simulink model "SimulinkBallBallancingBeam(EA)"  (R2019b)
settings: Solver=FixedStepAuto  StartTime=0.0  StopTime=10  RelTol=1e-3  EnableMultiTasking=on
values from neighbouring files (symbols this model uses):
  d = 0.05    [BallBallancingBeam(EA).m]    (also in System_Parameters.m; TransferFunction.m)
  g = -9.81    [BallBallancingBeam(EA).m]    (also in System_Parameters.m; TransferFunction.m)
  J = 6.3e-7    (= 6.3e-07)    [BallBallancingBeam(EA).m]    (also in System_Parameters.m = 6.2e-07; TransferFunction.m = 6.2e-07)
  L = .4    (= 0.4)    [BallBallancingBeam(EA).m]    (also in System_Parameters.m = 0.2; TransferFunction.m = 0.2)
  m = 0.0027    [BallBallancingBeam(EA).m]    (also in System_Parameters.m; TransferFunction.m)
  R = 0.02    [BallBallancingBeam(EA).m]    (also in System_Parameters.m = 0.0201; TransferFunction.m = 0.0201)
libraries: arduinolib x4, simulink x2, arduinosensorlib x1
settings Model: SILPILModeSetting=veronly  ExtModeTrigDuration=2  Creator=erika  LastModifiedBy=erika
settings SolverCC: PositivePriorityOrder=on
settings OptimizationCC: BufferReuse=off  EnhancedBackFolding=on  PassReuseOutputArgsAs=Individual arguments  ZeroExternalMemoryAtStartup=off  ZeroInternalMemoryAtStartup=off  MaxStackSize=64  OptimizeBlockOrder=speed  DifferentSizesBufferReuse=on  EfficientTunableParamExpr=on
settings DebuggingCC: ParameterTunabilityLossMsg=error  InitInArrayFormatMsg=none
settings HardwareCC: ProdBitPerInt=16  ProdBitPerPointer=16  ProdBitPerSizeT=16  ProdBitPerPtrDiffT=16  ProdLargestAtomicFloat=None  ProdWordSize=8  ProdHWDeviceType=Atmel->AVR  UseEmbeddedCoderFeatures=off
settings ModelReferenceCC: ModelReferenceNumInstancesAllowed=Single
settings SFSimCC: MATLABDynamicMemAlloc=off
settings RTWCC: SystemTargetFile=ert.tlc  HardwareBoard=Arduino Mega 2560  TLCOptions=-aInlineSetEventsForThisBaseRateFcn=TLC_FALSE -aSuppressMultiTaskScheduler=TLC_FALSE -aRateBasedStepFcn=1  TemplateMakefile=ert_default_tmf  GenerateReport=on  Toolchain=Arduino AVR  BuildConfiguration=Faster Runs  IncludeHyperlinkInReport=on  LaunchReport=on  GenerateTraceInfo=on  GenerateTraceReport=on  GenerateTraceReportSl=on  GenerateTraceReportSf=on  GenerateTraceReportEml=on
settings CodeAppCC: ForceParamTrailComments=on  IgnoreCustomStorageClasses=off  OperatorAnnotations=on  SimulinkDataObjDesc=on  SFDataObjDesc=on  InsertBlockDesc=on
settings ERTTargetCC: SupportContinuousTime=on  SupportNonInlinedSFcns=on  SupportVariableSizeSignals=on  ExtModeStaticAllocSize=2048

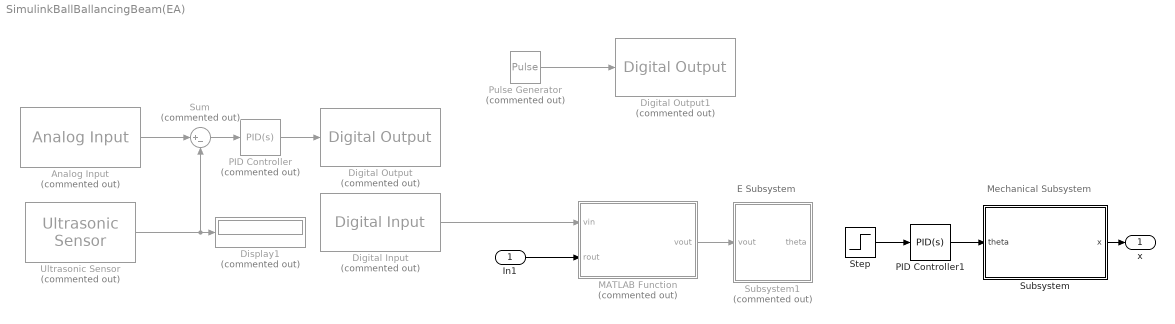
== system SimulinkBallBallancingBeam(EA) ==
  note: Mechanical Subsystem
  note: E Subsystem
  In1 : Inport  OutMin=[0]  OutMax=[5]
  Analog Input : arduinolib/Analog Input  Commented=on  pinNumber=4  ReadResultsOnly=off  ConversionTriggerSource=Software  ExternalTriggerType=uint32(0)  OutputDataType=uint16  EnableConversionCompleteNotify=off  EnableOuputStatus=off  SampleTime=-1  blockPlatform=arduino
  Digital Input : arduinolib/Digital Input  Commented=on  pinNumber=9  SampleTime=-1  blockPlatform=arduino
      settings: SourceProductName=Simulink Support Package for Arduino Hardware
  Digital Output : arduinolib/Digital Output  Commented=on  pinNumber=9  blockPlatform=arduino
  Digital Output1 : arduinolib/Digital Output  Commented=on  pinNumber=13  blockPlatform=arduino
  Display1 : Display  Commented=on
  MATLAB Function : MATLAB Function  Commented=on  TreatAsAtomicUnit=on
  PID Controller : simulink/Continuous/PID Controller  Commented=on  Controller=PID  Form=Parallel  TimeDomain=Continuous-time  SampleTime=-1  IntegratorMethod=Forward Euler  FilterMethod=Forward Euler  ControllerParametersSource=internal  P=2.5  I=0  D=1  UseFilter=on  N=100  TunerSelectOption=Transfer Function Based (PID Tuner App)  InitialConditionSource=internal  InitialConditionForIntegrator=0  InitialConditionForFilter=0  DifferentiatorICPrevScaledInput=0  ExternalReset=none  TrackingMode=off  Kt=1  LimitOutput=off  UpperSaturationLimit=inf  LowerSaturationLimit=-inf  LinearizeAsGain=on  AntiWindupMode=none  Kb=1  POutMin=[]  POutMax=[]  IOutMin=[]  IOutMax=[]  DOutMin=[]  DOutMax=[]  NOutMin=[]  NOutMax=[]  SumOutMin=[]  SumOutMax=[]  SaturationOutMin=[]  SaturationOutMax=[]  PParamMin=[]  PParamMax=[]  IParamMin=[]  IParamMax=[]  DParamMin=[]  DParamMax=[]  NParamMin=[]  NParamMax=[]  KbParamMin=[]  KbParamMax=[]  KtParamMin=[]  KtParamMax=[]  KbOutMin=[]  KbOutMax=[]  KtOutMin=[]  KtOutMax=[]  IntegratorOutMin=[]  IntegratorOutMax=[]  FilterOutMin=[]  FilterOutMax=[]  SumI1OutMin=[]  SumI1OutMax=[]  SumI2OutMin=[]  SumI2OutMax=[]  SumI3OutMin=[]  SumI3OutMax=[]  SumI4OutMin=[]  SumI4OutMax=[]  SumDOutMin=[]  SumDOutMax=[]  DifferentiatorOutMin=[]  DifferentiatorOutMax=[]  FilterDiffOutCoefMin=[]  FilterDiffOutCoefMax=[]  ReciprocalOutMin=[]  ReciprocalOutMax=[]  SumDenOutMin=[]  SumDenOutMax=[]  SumNumOutMin=[]  SumNumOutMax=[]  DivideOutMin=[]  DivideOutMax=[]  IntegratorContinuousStateAttributes=''  IntegratorStateMustResolveToSignalObject=off  IntegratorRTWStateStorageClass=Auto  FilterContinuousStateAttributes=''  FilterStateMustResolveToSignalObject=off  FilterRTWStateStorageClass=Auto  ParallelPVariant=InternalParameters  IdealPVariant=Disabled  IVariant=InternalParameters  DVariant=InternalParameters  IntegratorVariant=Continuous  SatVariant=Disabled  AWVariant=Passthrough  PCopyVariant=Disabled  TRVariant=Disabled  FdbkBlocksVariant=Forward  IdealPFdbkVariant=Disabled  SatFdbkVariant=Disabled  DerivativeFilterVariant=ContFilter  NVariant=InternalParameters  NCopyVariant=Disabled  FilterICVariant=InternalICsFilter  IntegratorICVariant=InternalICs  ExternalResetVariant=Disabled  TRSumVariant=Passthrough  SumFdbkVariant=Disabled  SumVariant=Sum_PID
  PID Controller1 : simulink/Continuous/PID Controller  Controller=PID  Form=Parallel  TimeDomain=Continuous-time  SampleTime=-1  IntegratorMethod=Forward Euler  FilterMethod=Forward Euler  ControllerParametersSource=internal  P=1  I=1  D=0  UseFilter=on  N=100  TunerSelectOption=Transfer Function Based (PID Tuner App)  InitialConditionSource=internal  InitialConditionForIntegrator=0  InitialConditionForFilter=0  DifferentiatorICPrevScaledInput=0  ExternalReset=none  TrackingMode=off  Kt=1  LimitOutput=off  UpperSaturationLimit=inf  LowerSaturationLimit=-inf  LinearizeAsGain=on  AntiWindupMode=none  Kb=1  POutMin=[]  POutMax=[]  IOutMin=[]  IOutMax=[]  DOutMin=[]  DOutMax=[]  NOutMin=[]  NOutMax=[]  SumOutMin=[]  SumOutMax=[]  SaturationOutMin=[]  SaturationOutMax=[]  PParamMin=[]  PParamMax=[]  IParamMin=[]  IParamMax=[]  DParamMin=[]  DParamMax=[]  NParamMin=[]  NParamMax=[]  KbParamMin=[]  KbParamMax=[]  KtParamMin=[]  KtParamMax=[]  KbOutMin=[]  KbOutMax=[]  KtOutMin=[]  KtOutMax=[]  IntegratorOutMin=[]  IntegratorOutMax=[]  FilterOutMin=[]  FilterOutMax=[]  SumI1OutMin=[]  SumI1OutMax=[]  SumI2OutMin=[]  SumI2OutMax=[]  SumI3OutMin=[]  SumI3OutMax=[]  SumI4OutMin=[]  SumI4OutMax=[]  SumDOutMin=[]  SumDOutMax=[]  DifferentiatorOutMin=[]  DifferentiatorOutMax=[]  FilterDiffOutCoefMin=[]  FilterDiffOutCoefMax=[]  ReciprocalOutMin=[]  ReciprocalOutMax=[]  SumDenOutMin=[]  SumDenOutMax=[]  SumNumOutMin=[]  SumNumOutMax=[]  DivideOutMin=[]  DivideOutMax=[]  IntegratorContinuousStateAttributes=''  IntegratorStateMustResolveToSignalObject=off  IntegratorRTWStateStorageClass=Auto  FilterContinuousStateAttributes=''  FilterStateMustResolveToSignalObject=off  FilterRTWStateStorageClass=Auto  ParallelPVariant=InternalParameters  IdealPVariant=Disabled  IVariant=InternalParameters  DVariant=InternalParameters  IntegratorVariant=Continuous  SatVariant=Disabled  AWVariant=Passthrough  PCopyVariant=Disabled  TRVariant=Disabled  FdbkBlocksVariant=Forward  IdealPFdbkVariant=Disabled  SatFdbkVariant=Disabled  DerivativeFilterVariant=ContFilter  NVariant=InternalParameters  NCopyVariant=Disabled  FilterICVariant=InternalICsFilter  IntegratorICVariant=InternalICs  ExternalResetVariant=Disabled  TRSumVariant=Passthrough  SumFdbkVariant=Disabled  SumVariant=Sum_PID
  Pulse Generator : DiscretePulseGenerator  Commented=on  Period=10  PulseWidth=5  SampleTime=0.1
  Step : Step  SampleTime=0
  Subsystem : Subsystem
  Subsystem1 : Subsystem  Commented=on
  Sum : Sum  Commented=on  Inputs=|+-
  Ultrasonic Sensor : arduinosensorlib/Ultrasonic Sensor  Commented=on  NumSignalPins=2  TrigPin=7  EchoPin=6  SignalPin=3  SampleTime_=0.1  blockPlatform=ARDUINO
      settings: SourceProductName=Simulink Support Package for Arduino Hardware  SourceProductBaseCode=ARDUINO
  x : Outport
  wires:
  In1/1 -> MATLAB Function/2(rout)
  Subsystem/1(x) -> x/1
  MATLAB Function/1(vout) -> Subsystem1/1("vout ")
  Pulse Generator/1 -> Digital Output1/1
  PID Controller/1 -> Digital Output/1
  Sum/1 -> PID Controller/1
  Digital Input/1 -> MATLAB Function/1(vin)
  Analog Input/1 -> Sum/1
  Ultrasonic Sensor/1 -> Sum/2, Display1/1
  PID Controller1/1 -> Subsystem/1(theta)
  Step/1 -> PID Controller1/1

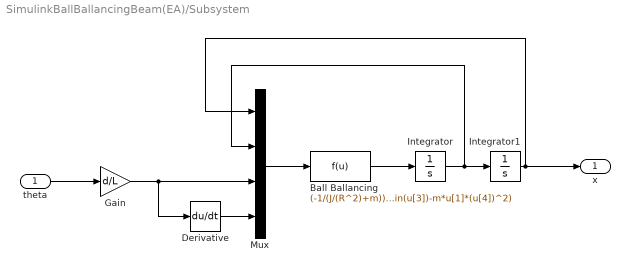
== system SimulinkBallBallancingBeam(EA)/Subsystem ==
  theta : Inport
  Ball Ballancing : Fcn  Expr=(-1/(J/(R^2)+m))*(m*g*sin(u[3])-m*u[1]*(u[4])^2)
  Derivative : Derivative
  Gain : Gain  Gain=d/L
  Integrator : Integrator
  Integrator1 : Integrator
  Mux : Mux
  x : Outport
  wires:
  Mux/1 -> Ball Ballancing/1
  Integrator1/1 -> x/1, Mux/1
  Gain/1 -> Derivative/1, Mux/3
  theta/1 -> Gain/1
  Integrator/1 -> Mux/2, Integrator1/1
  Ball Ballancing/1 -> Integrator/1
  Derivative/1 -> Mux/4

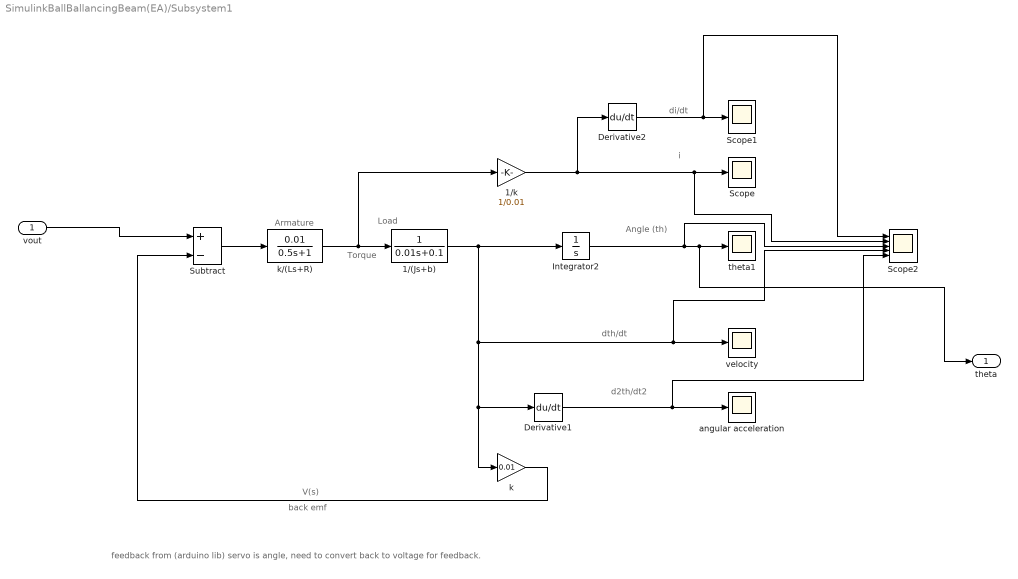
== system SimulinkBallBallancingBeam(EA)/Subsystem1 ==
  note: feedback from (arduino lib) servo is angle, need to convert back to voltage for feedback.
  note: Load
  note: back emf
  note: d2th/dt2
  note: V(s)
  note: Armature
  note: Torque
  note: i
  note: Angle (th)
  note: dth/dt
  note: di/dt
  "vout " : Inport
  1/(Js+b) : TransferFcn  Denominator=[0.01 0.1]
  1/k : Gain  Gain=1/0.01
  Derivative1 : Derivative
  Derivative2 : Derivative
  Integrator2 : Integrator
  Scope : Scope
  Scope1 : Scope
  Scope2 : Scope  NumInputPorts=5
  Subtract : Sum  Inputs=+-
  angular acceleration : Scope
  k : Gain  Gain=0.01
  k/(Ls+R) : TransferFcn  Numerator=[0.01]  Denominator=[0.5 1]
  theta1 : Scope
  velocity : Scope
  theta : Outport
  wires:
  Integrator2/1 -> Scope2/3, theta/1, theta1/1
  k/1 -> Subtract/2
  1/(Js+b)/1 -> k/1, Derivative1/1, Scope2/4, velocity/1, Integrator2/1
  k/(Ls+R)/1 -> 1/(Js+b)/1, 1/k/1
  Derivative2/1 -> Scope2/1, Scope1/1
  Subtract/1 -> k/(Ls+R)/1
  "vout "/1 -> Subtract/1
  Derivative1/1 -> Scope2/5, angular acceleration/1
  1/k/1 -> Derivative2/1, Scope2/2, Scope/1

== matlab function SimulinkBallBallancingBeam(EA)/MATLAB Function ==
  data: vin input; vout output; rout input
function vout = linmap(vin,rout)
% function for linear mapping between two ranges
% inputs:
% vin: the input vector you want to map, range [min(vin),max(vin)]
% rout: the range of the resulting vector
% output:
% vout: the resulting vector in range rout
% usage:
% >> v1 = linspace(-2,9,100);
% >> v2 = linmap(v1,[-5,5]);
%
a = min(vin);
b = max(vin);
c = rout(1);
d = rout(2);
vout = ((c+d) + (d-c)*((2*vin - (a+b))/(b-a)))/2;
endfunction y = fcn(u)

y = u;
